simulink model "CF009A_GmOvrlStMgr"  (R2013b)
settings: Solver=FixedStepDiscrete  SolverMode=SingleTasking  StartTime=0.0  StopTime=1  FixedStep=0.002  RelTol=1e-3
values from neighbouring files (symbols this model uses):
  APASTACTV_CNT_U08 = DataDict.Constant    [CF009A_GmOvrlStMgr_DataDict.m]
  APASTCTRLAVL_CNT_U08 = DataDict.Constant    [CF009A_GmOvrlStMgr_DataDict.m]
  ARCHGLBPRM_2MILLISEC_SEC_F32 = DataDict.Constant    [CF009A_GmOvrlStMgr_DataDict.m]
  GmOvrlStMgrApaHwTqThd = DataDict.Calibration    [CF009A_GmOvrlStMgr_DataDict.m]
  GmOvrlStMgrApaHwTqTiThd = DataDict.Calibration    [CF009A_GmOvrlStMgr_DataDict.m]
  GmOvrlStMgrApaMfgEna = DataDict.Calibration    [CF009A_GmOvrlStMgr_DataDict.m]
  GmOvrlStMgrEscMfgEna = DataDict.Calibration    [CF009A_GmOvrlStMgr_DataDict.m]
  GmOvrlStMgrHaptcAmp = DataDict.Calibration    [CF009A_GmOvrlStMgr_DataDict.m]
  GmOvrlStMgrHaptcDurn = DataDict.Calibration    [CF009A_GmOvrlStMgr_DataDict.m]
  GmOvrlStMgrHaptcFrq = DataDict.Calibration    [CF009A_GmOvrlStMgr_DataDict.m]
  GmOvrlStMgrHaptcReactnTi = DataDict.Calibration    [CF009A_GmOvrlStMgr_DataDict.m]
  GmOvrlStMgrHaptcReqTiThd = DataDict.Calibration    [CF009A_GmOvrlStMgr_DataDict.m]
  GmOvrlStMgrHwAgTarLimr = DataDict.Calibration    [CF009A_GmOvrlStMgr_DataDict.m]
  GmOvrlStMgrLkaHwTqThd1 = DataDict.Calibration    [CF009A_GmOvrlStMgr_DataDict.m]
  GmOvrlStMgrLkaHwTqThd2 = DataDict.Calibration    [CF009A_GmOvrlStMgr_DataDict.m]
  GmOvrlStMgrLkaHwTqTiThd1 = DataDict.Calibration    [CF009A_GmOvrlStMgr_DataDict.m]
  GmOvrlStMgrLkaHwTqTiThd2 = DataDict.Calibration    [CF009A_GmOvrlStMgr_DataDict.m]
  GmOvrlStMgrLkaMfgEna = DataDict.Calibration    [CF009A_GmOvrlStMgr_DataDict.m]
  GmOvrlStMgrLoaMtgtnHaptcFbOffTi = DataDict.Calibration    [CF009A_GmOvrlStMgr_DataDict.m]
  GmOvrlStMgrLoaMtgtnHaptcFbOnTi = DataDict.Calibration    [CF009A_GmOvrlStMgr_DataDict.m]
  GmOvrlStMgrLoaMtgtnHaptcFbStrtOnTi = DataDict.Calibration    [CF009A_GmOvrlStMgr_DataDict.m]
  GmOvrlStMgrLoaMtgtnHaptcFbTqMax = DataDict.Calibration    [CF009A_GmOvrlStMgr_DataDict.m]
  GmOvrlStMgrLoaMtgtnHaptcFbTqMin = DataDict.Calibration    [CF009A_GmOvrlStMgr_DataDict.m]
  GmOvrlStMgrLoaMtgtnHaptcFbVehSpdMax = DataDict.Calibration    [CF009A_GmOvrlStMgr_DataDict.m]
  GmOvrlStMgrLoaMtgtnHaptcFbVehSpdMin = DataDict.Calibration    [CF009A_GmOvrlStMgr_DataDict.m]
  GmOvrlStMgrLoaMtgtnHaptcFrq = DataDict.Calibration    [CF009A_GmOvrlStMgr_DataDict.m]
  GmOvrlStMgrLoaMtgtnStrtHaptcAmp = DataDict.Calibration    [CF009A_GmOvrlStMgr_DataDict.m]
  GmOvrlStMgrLoaStIgnCntrThd = DataDict.Calibration    [CF009A_GmOvrlStMgr_DataDict.m]
  GmOvrlStMgrShiftLvrTiThd = DataDict.Calibration    [CF009A_GmOvrlStMgr_DataDict.m]
  GmOvrlStMgrStandStillThd = DataDict.Calibration    [CF009A_GmOvrlStMgr_DataDict.m]
  GmOvrlStMgrStandStillTiThd = DataDict.Calibration    [CF009A_GmOvrlStMgr_DataDict.m]
  HAPTCSTACTV_CNT_U08 = DataDict.Constant    [CF009A_GmOvrlStMgr_DataDict.m]
  HAPTCSTWAIT_CNT_U08 = DataDict.Constant    [CF009A_GmOvrlStMgr_DataDict.m]
  HWOSCNFRQMIN_HZ_F32 = DataDict.Constant    [CF009A_GmOvrlStMgr_DataDict.m]
  LKAFLTCNTRTHD_CNT_U08 = DataDict.Constant    [CF009A_GmOvrlStMgr_DataDict.m]
  LKAFLTTMRTHD_MILLISEC_U32 = DataDict.Constant    [CF009A_GmOvrlStMgr_DataDict.m]
  LKASTPRMNTFAILD_CNT_U08 = DataDict.Constant    [CF009A_GmOvrlStMgr_DataDict.m]
  LoaMtgtnThdExcdd = DataDict.NTC    [CF009A_GmOvrlStMgr_DataDict.m]
  MILLISECTO100MICROSECCNVN_CNT_U32 = DataDict.Constant    [CF009A_GmOvrlStMgr_DataDict.m]
  NODEBSTEP_CNT_U16 = DataDict.Constant    [CF009A_GmOvrlStMgr_DataDict.m]
undefined symbols (not defined in the file or in its folder): LoaSt1, NtcSts1, NVM_RequestResultType, SysSt1
libraries: simulink x13, Fil x6, NxtrNvM x4, NxtrLim x4, NxtrAbslt x3, NxtrSign x2, FixdToFloat x1, FloatToFixd x1, LnrIntrpn x1
(part 3 of 8)

== system CF009A_GmOvrlStMgr/GmOvrlStMgr/GmOvrlStMgrPer1/HwTqFildIntlChk ==
  In1 : Inport
  Abslt_f32_f32 : NxtrAbslt/Abslt_f32_f32  SFunctionSpec=single y1 = Abslt_f32_f32(single u1)
      settings: AttributesFormatString=%<Name>
  CopyRight2 : Subsystem  Description=|  mask(Copyright Information){none=on}
      | Copyright info block.                                               
      |                                                                     
      | Place copyright information at the top of every subsystem in design.
      mask prompts: none "No parameters"
      mask help: Place copyright information at the top of every subsystem in design.
      mask Display:
      | NxtrConf = 'Nexteer Confidential';
      | 
      | sys = bdroot; %handle for the current model ("system")
      | first = get_param(sys,'Created');
      | first = first(end-3:end);  %year is last four digits
      | 
      | last = get_param(sys,'LastModifiedDate');
      | if isempty(last)
      |     last = datestr(now,'yyyy');
      | else
      |     last = last(end-3:end);
      | end
      | 
      | if strcmp(first,last)
      |     fprintf('%s -- Copyright %s Nexteer',NxtrConf,first)
      | else
      |     fprintf('%s -- %s%s- %s Nexteer',NxtrConf,char(169),first,last)
      | end
  FilLpUpdOutp : Fil/FilLpUpdOutp  StVar=HwTqOscnLpFil
      settings: AttributesFormatString=StVar: %<StVar>
  Interval Test4 : simulink/Logic and Bit Operations/Interval Test  IntervalClosedRight=on  uplimit=GmOvrlStMgrLoaMtgtnHaptcFbTqMax  IntervalClosedLeft=on  lowlimit=GmOvrlStMgrLoaMtgtnHaptcFbTqMin  OutDataTypeStr=boolean
  Out1 : Outport
  wires:
  Interval Test4/1 -> Out1/1
  Abslt_f32_f32/1 -> Interval Test4/1
  FilLpUpdOutp/1 -> Abslt_f32_f32/1
  In1/1 -> FilLpUpdOutp/1

== system CF009A_GmOvrlStMgr/GmOvrlStMgr/GmOvrlStMgrPer1/Inct_IgnCntr_Once ==
  IgnCntrLcl : Inport  RequirementInfo={} %GIDa_31be0032_d248_4158_b577_634f04f9b9d9
  Action Port : ActionPort  ActionType=then
  CopyRight2 : Subsystem  Description=|  mask(Copyright Information){none=on}
      | Copyright info block.                                               
      |                                                                     
      | Place copyright information at the top of every subsystem in design.
      mask prompts: none "No parameters"
      mask help: Place copyright information at the top of every subsystem in design.
      mask Display:
      | NxtrConf = 'Nexteer Confidential';
      | 
      | sys = bdroot; %handle for the current model ("system")
      | first = get_param(sys,'Created');
      | if(isempty(first))
      |     first = datestr(now,'yyyy');
      | else
      |     first = first(end-3:end);  %year is last four digits
      | end
      | 
      | last = get_param(sys,'LastModifiedDate');
      | if isempty(last)
      |     last = datestr(now,'yyyy');
      | else
      |     last = last(end-3:end);
      | end
      | 
      | if strcmp(first,last)
      |     fprintf('%s -- Copyright %s Nexteer',NxtrConf,first)
      | else
      |     fprintf('%s -- %s%s- %s Nexteer',NxtrConf,char(169),first,last)
      | end
  Data Store Read1 : DataStoreRead  DataStoreName=IgnCntrUpd
  If20 : If  IfExpression=~u1  ShowElse=off
  IgnCntr : Subsystem  TreatAsAtomicUnit=on
  wires:
  If20/1 -> IgnCntr/Action
  Data Store Read1/1 -> If20/1
  IgnCntrLcl/1 -> IgnCntr/1(IgnCntrLcl)

== system CF009A_GmOvrlStMgr/GmOvrlStMgr/GmOvrlStMgrPer1/LKAIntv ==
  note: To Determine if the driver is opposing the LKA command
  HwTq : Inport
  LkaTqCmdCdnd : Inport  Port=2
  Abslt_f32_f32 : NxtrAbslt/Abslt_f32_f32  SFunctionSpec=single y1 = Abslt_f32_f32(single u1)
      settings: AttributesFormatString=%<Name>
  CopyRight2 : Subsystem  Description=|  mask(Copyright Information){none=on}
      | Copyright info block.                                               
      |                                                                     
      | Place copyright information at the top of every subsystem in design.
      mask prompts: none "No parameters"
      mask help: Place copyright information at the top of every subsystem in design.
      mask Display:
      | NxtrConf = 'Nexteer Confidential';
      | 
      | sys = bdroot; %handle for the current model ("system")
      | first = get_param(sys,'Created');
      | first = first(end-3:end);  %year is last four digits
      | 
      | last = get_param(sys,'LastModifiedDate');
      | if isempty(last)
      |     last = datestr(now,'yyyy');
      | else
      |     last = last(end-3:end);
      | end
      | 
      | if strcmp(first,last)
      |     fprintf('%s -- Copyright %s Nexteer',NxtrConf,first)
      | else
      |     fprintf('%s -- %s%s- %s Nexteer',NxtrConf,char(169),first,last)
      | end
  Data Store Write1 : DataStoreWrite  DataStoreName=LkaIntvPrev
  FilLpUpdOutp : Fil/FilLpUpdOutp  StVar=HwTqLkaLpFil
      settings: AttributesFormatString=StVar: %<StVar>
  HwTqLkaTqSignEqu : Subsystem  TreatAsAtomicUnit=on
  HwTqLkaTqSignNotEqu : Subsystem  TreatAsAtomicUnit=on
  If2 : If  IfExpression=u1
  Merge3 : Merge
  Relational Operator : RelationalOperator  Operator===  OutDataTypeStr=boolean
  Sign_s08_f1 : NxtrSign/Sign_s08_f32  SFunctionSpec=int8 y1 = Sign_s08_f32(single u1)
  Sign_s08_f32 : NxtrSign/Sign_s08_f32  SFunctionSpec=int8 y1 = Sign_s08_f32(single u1)
  LKAIntv : Outport
  wires:
  [HwTq] -> Sign_s08_f1/1
  FilLpUpdOutp/1 -> Abslt_f32_f32/1
  LkaTqCmdCdnd/1 -> Sign_s08_f32/1
  Sign_s08_f32/1 -> Relational Operator/2
  Sign_s08_f1/1 -> Relational Operator/1
  Relational Operator/1 -> If2/1
  If2/1 -> HwTqLkaTqSignEqu/Action
  If2/2 -> HwTqLkaTqSignNotEqu/Action
  Abslt_f32_f32/1 -> [AbsHwTqFild]
  HwTq/1 -> [HwTq], FilLpUpdOutp/1
  [AbsHwTqFild] -> HwTqLkaTqSignNotEqu/1(AbsHwTqFild)
  HwTqLkaTqSignEqu/1(LKAIntv) -> Merge3/1
  HwTqLkaTqSignNotEqu/1(LKAIntv) -> Merge3/2
  Merge3/1 -> Data Store Write1/1, LKAIntv/1

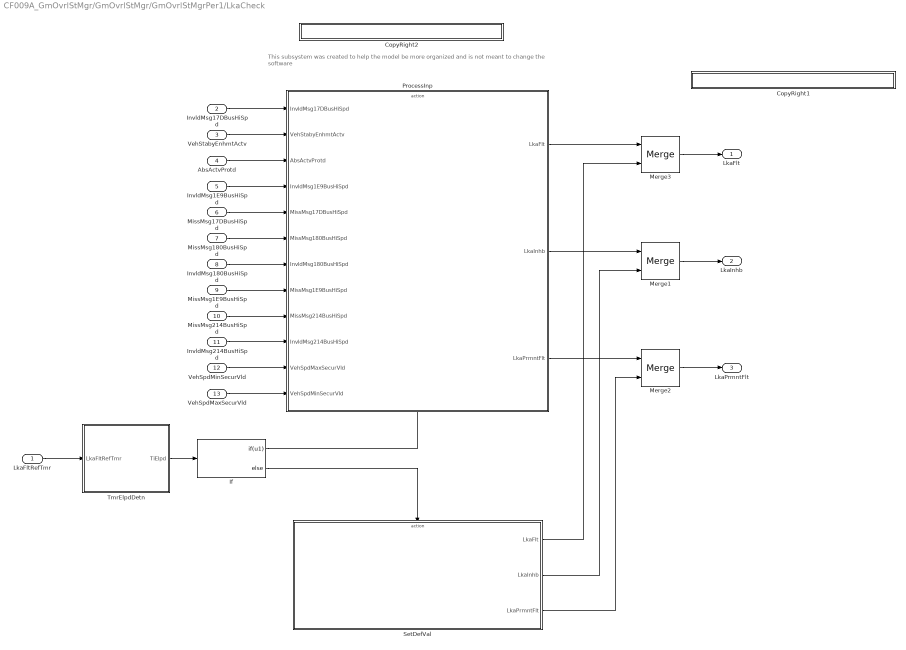
== system CF009A_GmOvrlStMgr/GmOvrlStMgr/GmOvrlStMgrPer1/LkaCheck ==
  note: This subsystem was created to help the model be more organized and is not meant to change the software
  LkaFltRefTmr : Inport
  InvldMsg17DBusHiSpd : Inport  RequirementInfo={} %GIDa_2e808d10_eb15_4dce_ab7e_f3136c3c94f9  Port=2
  VehStabyEnhmtActv : Inport  RequirementInfo={} %GIDa_3591af50_b788_48cc_aa03_0dae07c6844d  Port=3
  AbsActvProtd : Inport  RequirementInfo={} %GIDa_a71630fb_1116_4598_9016_42ba8f18e277  Port=4
  InvldMsg1E9BusHiSpd : Inport  RequirementInfo={} %GIDa_44549ea5_d3bf_44aa_ad01_370864df879b  Port=5
  MissMsg17DBusHiSpd : Inport  RequirementInfo={} %GIDa_3510a1c9_681a_4837_901b_d1fdb7257903  Port=6
  MissMsg180BusHiSpd : Inport  RequirementInfo={} %GIDa_29db47c2_2496_45a5_a94f_ca81858af381  Port=7
  InvldMsg180BusHiSpd : Inport  RequirementInfo={} %GIDa_c95a73a8_1984_48d0_982e_2a99b56d2733  Port=8
  MissMsg1E9BusHiSpd : Inport  RequirementInfo={} %GIDa_8896b252_879d_4242_80a0_160e6dd0973f  Port=9
  MissMsg214BusHiSpd : Inport  RequirementInfo={} %GIDa_e93b804e_26b6_4a26_9fbc_29131c435554  Port=10
  InvldMsg214BusHiSpd : Inport  RequirementInfo={} %GIDa_23b949d5_a203_4809_9d67_db82e22a32ce  Port=11
  VehSpdMinSecurVld : Inport  Port=12
  VehSpdMaxSecurVld : Inport  Port=13
  CopyRight1 : Subsystem  Description=|  mask(Copyright Information){none=on}
      | Copyright info block.                                               
      |                                                                     
      | Place copyright information at the top of every subsystem in design.
      mask prompts: none "No parameters"
      mask help: Place copyright information at the top of every subsystem in design.
      mask Display:
      | NxtrConf = 'Nexteer Confidential';
      | 
      | sys = bdroot; %handle for the current model ("system")
      | first = get_param(sys,'Created');
      | if(isempty(first))
      |     first = datestr(now,'yyyy');
      | else
      |     first = first(end-3:end);  %year is last four digits
      | end
      | 
      | last = get_param(sys,'LastModifiedDate');
      | if isempty(last)
      |     last = datestr(now,'yyyy');
      | else
      |     last = last(end-3:end);
      | end
      | 
      | if strcmp(first,last)
      |     fprintf('%s -- Copyright %s Nexteer',NxtrConf,first)
      | else
      |     fprintf('%s -- %s%s- %s Nexteer',NxtrConf,char(169),first,last)
      | end
  CopyRight2 : Subsystem  Description=|  mask(Copyright Information){none=on}
      | Copyright info block.                                               
      |                                                                     
      | Place copyright information at the top of every subsystem in design.
      mask prompts: none "No parameters"
      mask help: Place copyright information at the top of every subsystem in design.
      mask Display:
      | NxtrConf = 'Nexteer Confidential';
      | 
      | sys = bdroot; %handle for the current model ("system")
      | first = get_param(sys,'Created');
      | first = first(end-3:end);  %year is last four digits
      | 
      | last = get_param(sys,'LastModifiedDate');
      | if isempty(last)
      |     last = datestr(now,'yyyy');
      | else
      |     last = last(end-3:end);
      | end
      | 
      | if strcmp(first,last)
      |     fprintf('%s -- Copyright %s Nexteer',NxtrConf,first)
      | else
      |     fprintf('%s -- %s%s- %s Nexteer',NxtrConf,char(169),first,last)
      | end
  If : If  RequirementInfo={} %GIDa_1f091b25_2844_4bea_86d8_428600b90772  Priority=0  IfExpression=u1
  Merge1 : Merge  RequirementInfo={} %GIDa_91ec1541_edd6_4e63_a334_a58d5e1b75c9
  Merge2 : Merge  RequirementInfo={} %GIDa_1f0d8a4f_5d48_411b_8451_0a42805f8c5f
  Merge3 : Merge  RequirementInfo={} %GIDa_d55ab1e5_a42e_4154_95a8_1fe89e6aae2d
  ProcessInp : Subsystem  TreatAsAtomicUnit=on
  SetDefVal : Subsystem  TreatAsAtomicUnit=on
  TmrElpdDetn : Subsystem  RequirementInfo={} %GIDa_14aacf7e_b947_4f82_958b_883fcdf93c59  TreatAsAtomicUnit=on
  LkaFlt : Outport
  LkaInhb : Outport  Port=2
  LkaPrmntFlt : Outport  Port=3
  wires:
  LkaFltRefTmr/1 -> TmrElpdDetn/1(LkaFltRefTmr)
  TmrElpdDetn/1(TiElpd) -> If/1
  If/2 -> SetDefVal/Action
  If/1 -> ProcessInp/Action
  MissMsg17DBusHiSpd/1 -> ProcessInp/5(MissMsg17DBusHiSpd)
  MissMsg180BusHiSpd/1 -> ProcessInp/6(MissMsg180BusHiSpd)
  InvldMsg180BusHiSpd/1 -> ProcessInp/7(InvldMsg180BusHiSpd)
  MissMsg1E9BusHiSpd/1 -> ProcessInp/8(MissMsg1E9BusHiSpd)
  MissMsg214BusHiSpd/1 -> ProcessInp/9(MissMsg214BusHiSpd)
  InvldMsg214BusHiSpd/1 -> ProcessInp/10(InvldMsg214BusHiSpd)
  VehSpdMinSecurVld/1 -> ProcessInp/11(VehSpdMaxSecurVld)
  VehSpdMaxSecurVld/1 -> ProcessInp/12(VehSpdMinSecurVld)
  InvldMsg17DBusHiSpd/1 -> ProcessInp/1(InvldMsg17DBusHiSpd)
  VehStabyEnhmtActv/1 -> ProcessInp/2(VehStabyEnhmtActv)
  AbsActvProtd/1 -> ProcessInp/3(AbsActvProtd)
  InvldMsg1E9BusHiSpd/1 -> ProcessInp/4(InvldMsg1E9BusHiSpd)
  ProcessInp/1(LkaFlt) -> Merge3/1
  Merge3/1 -> LkaFlt/1
  Merge1/1 -> LkaInhb/1
  Merge2/1 -> LkaPrmntFlt/1
  SetDefVal/1(LkaFlt) -> Merge3/2
  ProcessInp/2(LkaInhb) -> Merge1/1
  SetDefVal/2(LkaInhb) -> Merge1/2
  ProcessInp/3(LkaPrmntFlt) -> Merge2/1
  SetDefVal/3(LkaPrmntFlt) -> Merge2/2

== system CF009A_GmOvrlStMgr/GmOvrlStMgr/GmOvrlStMgrPer1/LoaStLimdOrSwBasdMtgtn ==
  LoaSt : Inport
  CopyRight2 : Subsystem  Description=|  mask(Copyright Information){none=on}
      | Copyright info block.                                               
      |                                                                     
      | Place copyright information at the top of every subsystem in design.
      mask prompts: none "No parameters"
      mask help: Place copyright information at the top of every subsystem in design.
      mask Display:
      | NxtrConf = 'Nexteer Confidential';
      | 
      | sys = bdroot; %handle for the current model ("system")
      | first = get_param(sys,'Created');
      | if(isempty(first))
      |     first = datestr(now,'yyyy');
      | else
      |     first = first(end-3:end);  %year is last four digits
      | end
      | 
      | last = get_param(sys,'LastModifiedDate');
      | if isempty(last)
      |     last = datestr(now,'yyyy');
      | else
      |     last = last(end-3:end);
      | end
      | 
      | if strcmp(first,last)
      |     fprintf('%s -- Copyright %s Nexteer',NxtrConf,first)
      | else
      |     fprintf('%s -- %s%s- %s Nexteer',NxtrConf,char(169),first,last)
      | end
  Enumerated Constant : simulink/Sources/Enumerated Constant  OutDataTypeStr=Enum: LoaSt1  Value=LoaSt1.LOAST_LIMD  SampleTime=inf
  Enumerated Constant1 : simulink/Sources/Enumerated Constant  OutDataTypeStr=Enum: LoaSt1  Value=LoaSt1.LOAST_SWBASDMTGTN  SampleTime=inf
  If2 : If  IfExpression=u1
  Logical Operator5 : Logic  Operator=OR  AllPortsSameDT=off  OutDataTypeStr=boolean
  Merge : Merge
  Relational Operator2 : RelationalOperator  Operator===  OutDataTypeStr=boolean
  Relational Operator4 : RelationalOperator  Operator===  OutDataTypeStr=boolean
  Set_false_LoaStLimdOrSwBasdMtgtn : Subsystem
  Set_true_LoaStLimdOrSwBasdMtgtn : Subsystem
  LoaStLimdOrSwBasdMtgtn : Outport
  wires:
  Set_true_LoaStLimdOrSwBasdMtgtn/1(LoaStLimdOrSwBasdMtgtn) -> Merge/1
  If2/1 -> Set_true_LoaStLimdOrSwBasdMtgtn/Action
  Relational Operator4/1 -> Logical Operator5/2
  Enumerated Constant/1 -> Relational Operator2/1
  If2/2 -> Set_false_LoaStLimdOrSwBasdMtgtn/Action
  Enumerated Constant1/1 -> Relational Operator4/2
  LoaSt/1 -> Relational Operator4/1, Relational Operator2/2
  Logical Operator5/1 -> If2/1
  Relational Operator2/1 -> Logical Operator5/1
  Set_false_LoaStLimdOrSwBasdMtgtn/1(LoaStLimdOrSwBasdMtgtn) -> Merge/2
  Merge/1 -> LoaStLimdOrSwBasdMtgtn/1

== system CF009A_GmOvrlStMgr/GmOvrlStMgr/GmOvrlStMgrPer1/SysStNotOperate_TqOscnDi_AmpZero_FrqMin ==
  Action Port : ActionPort  ActionType=else
  Constant : Constant  Value=0  OutDataTypeStr=single
  Constant1 : Constant  Value=HWOSCNFRQMIN_HZ_F32  OutDataTypeStr=single
  Constant9 : Constant  Value=false  OutDataTypeStr=boolean
      settings: AttributesFormatString=%<OutDataTypeStr>
  CopyRight2 : Subsystem  Description=|  mask(Copyright Information){none=on}
      | Copyright info block.                                               
      |                                                                     
      | Place copyright information at the top of every subsystem in design.
      mask prompts: none "No parameters"
      mask help: Place copyright information at the top of every subsystem in design.
      mask Display:
      | NxtrConf = 'Nexteer Confidential';
      | 
      | sys = bdroot; %handle for the current model ("system")
      | first = get_param(sys,'Created');
      | if(isempty(first))
      |     first = datestr(now,'yyyy');
      | else
      |     first = first(end-3:end);  %year is last four digits
      | end
      | 
      | last = get_param(sys,'LastModifiedDate');
      | if isempty(last)
      |     last = datestr(now,'yyyy');
      | else
      |     last = last(end-3:end);
      | end
      | 
      | if strcmp(first,last)
      |     fprintf('%s -- Copyright %s Nexteer',NxtrConf,first)
      | else
      |     fprintf('%s -- %s%s- %s Nexteer',NxtrConf,char(169),first,last)
      | end
  HwOscnEna : Outport  RequirementInfo={} %GIDa_8ea3e658_ac34_4ba8_8bc0_f59fa217fe1b
  HwOscnMotAmp : Outport  RequirementInfo={} %GIDa_cab656c5_ad5b_40cd_9e56_00ba20adb2b9  Port=2
  HwOscnFrq : Outport  RequirementInfo={} %GIDa_8a1cbf52_fe7e_4d9e_a07e_11d275854390  Port=3
  wires:
  Constant9/1 -> HwOscnEna/1
  Constant/1 -> HwOscnMotAmp/1
  Constant1/1 -> HwOscnFrq/1

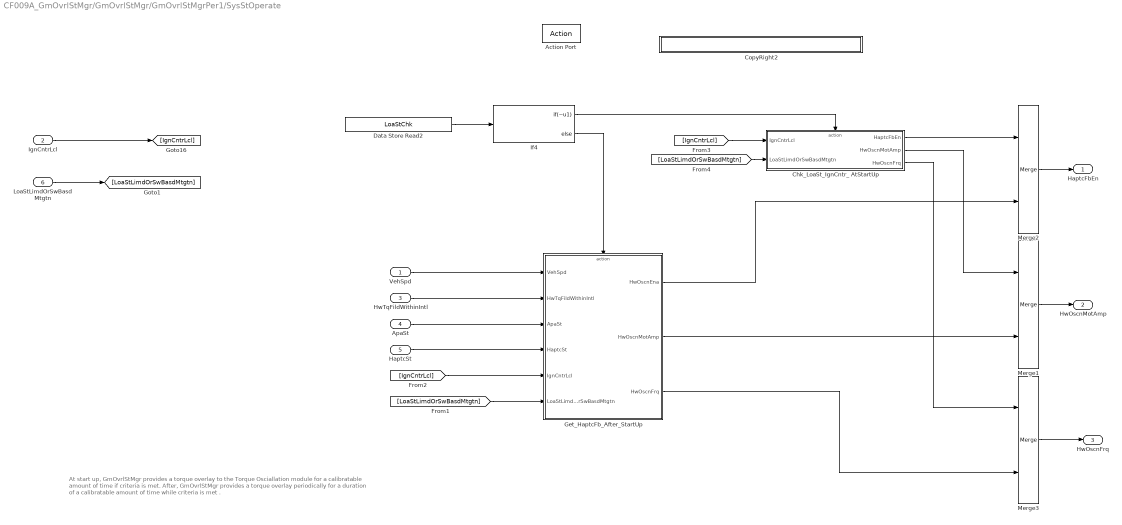
== system CF009A_GmOvrlStMgr/GmOvrlStMgr/GmOvrlStMgrPer1/SysStOperate ==
  note: At start up, GmOvrlStMgr provides a torque overlay to the Torque Osciallation module for a calibratable amount of time if criteria is met.
      | After, GmOvrlStMgr provides a torque overlay periodically for a duration of a calibratable amount of time while criteria is met .
  VehSpd : Inport  RequirementInfo={} %GIDa_2652915f_2b3a_4256_8b6a_592e4995acc0
  IgnCntrLcl : Inport  RequirementInfo={} %GIDa_e888d205_558d_4af3_99a0_723aa084dc2d  Port=2
  HwTqFildWithinIntl : Inport  RequirementInfo={} %GIDa_45987a6d_ef79_4fe8_8691_cf583e52523b  Port=3
  ApaSt : Inport  RequirementInfo={} %GIDa_af2c68b1_95b1_4974_8eec_dffb9414db10  Port=4
  HaptcSt : Inport  RequirementInfo={} %GIDa_9d2ea291_f891_4713_85e4_8f6b9ae44dd1  Port=5
  LoaStLimdOrSwBasdMtgtn : Inport  RequirementInfo={} %GIDa_9e2f6aad_f776_44c0_8c0b_e29e77d1c4aa  Port=6
  Action Port : ActionPort  ActionType=then
  Chk_LoaSt_IgnCntr_ AtStartUp : Subsystem  TreatAsAtomicUnit=on
  CopyRight2 : Subsystem  Description=|  mask(Copyright Information){none=on}
      | Copyright info block.                                               
      |                                                                     
      | Place copyright information at the top of every subsystem in design.
      mask prompts: none "No parameters"
      mask help: Place copyright information at the top of every subsystem in design.
      mask Display:
      | NxtrConf = 'Nexteer Confidential';
      | 
      | sys = bdroot; %handle for the current model ("system")
      | first = get_param(sys,'Created');
      | if(isempty(first))
      |     first = datestr(now,'yyyy');
      | else
      |     first = first(end-3:end);  %year is last four digits
      | end
      | 
      | last = get_param(sys,'LastModifiedDate');
      | if isempty(last)
      |     last = datestr(now,'yyyy');
      | else
      |     last = last(end-3:end);
      | end
      | 
      | if strcmp(first,last)
      |     fprintf('%s -- Copyright %s Nexteer',NxtrConf,first)
      | else
      |     fprintf('%s -- %s%s- %s Nexteer',NxtrConf,char(169),first,last)
      | end
  Data Store Read2 : DataStoreRead  DataStoreName=LoaStChk
  Get_HaptcFb_After_StartUp : Subsystem  TreatAsAtomicUnit=on
  If4 : If  IfExpression=~u1
  Merge1 : Merge
  Merge2 : Merge
  Merge3 : Merge
  HaptcFbEn : Outport
  HwOscnMotAmp : Outport  RequirementInfo={} %GIDa_30e263ba_ec21_46fb_a2a6_c50359a0704f  Port=2
  HwOscnFrq : Outport  RequirementInfo={} %GIDa_0a2b2e9b_0783_462d_9074_6b0e98e66f91  Port=3
  wires:
  Data Store Read2/1 -> If4/1
  If4/1 -> Chk_LoaSt_IgnCntr_ AtStartUp/Action
  If4/2 -> Get_HaptcFb_After_StartUp/Action
  Chk_LoaSt_IgnCntr_ AtStartUp/2(HwOscnMotAmp) -> Merge1/1
  Chk_LoaSt_IgnCntr_ AtStartUp/1(HaptcFbEn) -> Merge2/1
  Chk_LoaSt_IgnCntr_ AtStartUp/3(HwOscnFrq) -> Merge3/1
  Get_HaptcFb_After_StartUp/1(HwOscnEna) -> Merge2/2
  Get_HaptcFb_After_StartUp/3(HwOscnFrq) -> Merge3/2
  Get_HaptcFb_After_StartUp/2(HwOscnMotAmp) -> Merge1/2
  Merge2/1 -> HaptcFbEn/1
  Merge3/1 -> HwOscnFrq/1
  Merge1/1 -> HwOscnMotAmp/1
  VehSpd/1 -> Get_HaptcFb_After_StartUp/1(VehSpd)
  HwTqFildWithinIntl/1 -> Get_HaptcFb_After_StartUp/2(HwTqFildWithinIntl)
  ApaSt/1 -> Get_HaptcFb_After_StartUp/3(ApaSt)
  HaptcSt/1 -> Get_HaptcFb_After_StartUp/4(HaptcSt)
  IgnCntrLcl/1 -> [IgnCntrLcl]
  [IgnCntrLcl] -> Chk_LoaSt_IgnCntr_ AtStartUp/1(IgnCntrLcl)
  [IgnCntrLcl] -> Get_HaptcFb_After_StartUp/5(IgnCntrLcl)
  [LoaStLimdOrSwBasdMtgtn] -> Get_HaptcFb_After_StartUp/6(LoaStLimdOrSwBasdMtgtn)
  LoaStLimdOrSwBasdMtgtn/1 -> [LoaStLimdOrSwBasdMtgtn]
  [LoaStLimdOrSwBasdMtgtn] -> Chk_LoaSt_IgnCntr_ AtStartUp/2(LoaStLimdOrSwBasdMtgtn)

== system CF009A_GmOvrlStMgr/GmOvrlStMgr/GmOvrlStMgrPer1/Timer for HwHaptcEna ==
  Ena : Inport
  TiThd : Inport  Port=2
  Constant : Constant  Value=0  OutDataTypeStr=uint32
  Constant2 : Constant  Value=MILLISECTO100MICROSECCNVN_CNT_U32
  CopyRight2 : Subsystem  Description=|  mask(Copyright Information){none=on}
      | Copyright info block.                                               
      |                                                                     
      | Place copyright information at the top of every subsystem in design.
      mask prompts: none "No parameters"
      mask help: Place copyright information at the top of every subsystem in design.
      mask Display:
      | NxtrConf = 'Nexteer Confidential';
      | 
      | sys = bdroot; %handle for the current model ("system")
      | first = get_param(sys,'Created');
      | if(isempty(first))
      |     first = datestr(now,'yyyy');
      | else
      |     first = first(end-3:end);  %year is last four digits
      | end
      | 
      | last = get_param(sys,'LastModifiedDate');
      | if isempty(last)
      |     last = datestr(now,'yyyy');
      | else
      |     last = last(end-3:end);
      | end
      | 
      | if strcmp(first,last)
      |     fprintf('%s -- Copyright %s Nexteer',NxtrConf,first)
      | else
      |     fprintf('%s -- %s%s- %s Nexteer',NxtrConf,char(169),first,last)
      | end
  Data Store Read : DataStoreRead  Priority=1  DataStoreName=PrevHaptcReqEna
      settings: AttributesFormatString="Priority:  %<Priority>"
  Data Store Write1 : DataStoreWrite  Priority=2  DataStoreName=PrevHaptcReqEna
      settings: AttributesFormatString="Priority:  %<Priority>"
  If : If  NumInputs=2  IfExpression=u1&(~u2)  ElseIfExpressions=u1&u2
  If Action Subsystem : Subsystem  TreatAsAtomicUnit=on
  If Action Subsystem1 : Subsystem  TreatAsAtomicUnit=on
  If Action Subsystem2 : Subsystem  TreatAsAtomicUnit=on
  Merge : Merge  Inputs=3
  Product : Product
  Relational Operator3 : RelationalOperator  OutDataTypeStr=boolean
  Out1 : Outport
  wires:
  If Action Subsystem2/1(Out1) -> Merge/2
  If/2 -> If Action Subsystem2/Action
  Data Store Read/1 -> If/2
  Ena/1 -> If/1, Data Store Write1/1
  Relational Operator3/1 -> Out1/1
  Merge/1 -> Relational Operator3/1
  Product/1 -> Relational Operator3/2
  Constant2/1 -> Product/2
  TiThd/1 -> Product/1
  Constant/1 -> If Action Subsystem1/1(In1)
  If Action Subsystem1/1(Out1) -> Merge/3
  If Action Subsystem/1(Out) -> Merge/1
  If/3 -> If Action Subsystem1/Action
  If/1 -> If Action Subsystem/Action

== system CF009A_GmOvrlStMgr/GmOvrlStMgr/GmOvrlStMgrPer1/Timer for ShiftLvrRvs ==
  Ena : Inport
  TiThd : Inport  Port=2
  Constant : Constant  Value=0  OutDataTypeStr=uint32
  Constant2 : Constant  Value=MILLISECTO100MICROSECCNVN_CNT_U32
  CopyRight2 : Subsystem  Description=|  mask(Copyright Information){none=on}
      | Copyright info block.                                               
      |                                                                     
      | Place copyright information at the top of every subsystem in design.
      mask prompts: none "No parameters"
      mask help: Place copyright information at the top of every subsystem in design.
      mask Display:
      | NxtrConf = 'Nexteer Confidential';
      | 
      | sys = bdroot; %handle for the current model ("system")
      | first = get_param(sys,'Created');
      | first = first(end-3:end);  %year is last four digits
      | 
      | last = get_param(sys,'LastModifiedDate');
      | if isempty(last)
      |     last = datestr(now,'yyyy');
      | else
      |     last = last(end-3:end);
      | end
      | 
      | if strcmp(first,last)
      |     fprintf('%s -- Copyright %s Nexteer',NxtrConf,first)
      | else
      |     fprintf('%s -- %s%s- %s Nexteer',NxtrConf,char(169),first,last)
      | end
  Data Store Read : DataStoreRead  Priority=1  DataStoreName=PrevShiftLvrRvsEna
      settings: AttributesFormatString="priority:  %<Priority>"
  Data Store Write1 : DataStoreWrite  Priority=2  DataStoreName=PrevShiftLvrRvsEna
      settings: AttributesFormatString="priority:  %<Priority>"
  If : If  NumInputs=2  IfExpression=u1&(~u2)  ElseIfExpressions=u1&u2
  If Action Subsystem : Subsystem  TreatAsAtomicUnit=on
  If Action Subsystem1 : Subsystem  TreatAsAtomicUnit=on
  If Action Subsystem2 : Subsystem  TreatAsAtomicUnit=on
  Merge : Merge  Inputs=3
  Product : Product
  Relational Operator3 : RelationalOperator  OutDataTypeStr=boolean
  Out1 : Outport
  wires:
  If Action Subsystem2/1(Out) -> Merge/2
  If/2 -> If Action Subsystem2/Action
  Data Store Read/1 -> If/2
  Ena/1 -> If/1, Data Store Write1/1
  Relational Operator3/1 -> Out1/1
  Merge/1 -> Relational Operator3/1
  Product/1 -> Relational Operator3/2
  Constant2/1 -> Product/2
  TiThd/1 -> Product/1
  Constant/1 -> If Action Subsystem1/1(In1)
  If Action Subsystem1/1(Out1) -> Merge/3
  If Action Subsystem/1(Out) -> Merge/1
  If/3 -> If Action Subsystem1/Action
  If/1 -> If Action Subsystem/Action

== system CF009A_GmOvrlStMgr/GmOvrlStMgr/GmOvrlStMgrPer1/Timer for VehStandStill ==
  Ena : Inport
  TiThd : Inport  Port=2
  Constant : Constant  Value=0  OutDataTypeStr=uint32
  Constant2 : Constant  Value=MILLISECTO100MICROSECCNVN_CNT_U32
  CopyRight2 : Subsystem  Description=|  mask(Copyright Information){none=on}
      | Copyright info block.                                               
      |                                                                     
      | Place copyright information at the top of every subsystem in design.
      mask prompts: none "No parameters"
      mask help: Place copyright information at the top of every subsystem in design.
      mask Display:
      | NxtrConf = 'Nexteer Confidential';
      | 
      | sys = bdroot; %handle for the current model ("system")
      | first = get_param(sys,'Created');
      | first = first(end-3:end);  %year is last four digits
      | 
      | last = get_param(sys,'LastModifiedDate');
      | if isempty(last)
      |     last = datestr(now,'yyyy');
      | else
      |     last = last(end-3:end);
      | end
      | 
      | if strcmp(first,last)
      |     fprintf('%s -- Copyright %s Nexteer',NxtrConf,first)
      | else
      |     fprintf('%s -- %s%s- %s Nexteer',NxtrConf,char(169),first,last)
      | end
  Data Store Read : DataStoreRead  Priority=1  DataStoreName=PrevVehStandStillEna
      settings: AttributesFormatString="Priority:  %<Priority>"
  Data Store Write1 : DataStoreWrite  Priority=2  DataStoreName=PrevVehStandStillEna
      settings: AttributesFormatString="Priority:  %<Priority>"
  If : If  NumInputs=2  IfExpression=u1&(~u2)  ElseIfExpressions=u1&u2
  If Action Subsystem : Subsystem  TreatAsAtomicUnit=on
  If Action Subsystem1 : Subsystem  TreatAsAtomicUnit=on
  If Action Subsystem2 : Subsystem  TreatAsAtomicUnit=on
  Merge : Merge  Inputs=3
  Product : Product
  Relational Operator3 : RelationalOperator  OutDataTypeStr=boolean
  Out1 : Outport
  wires:
  If Action Subsystem2/1(Out1) -> Merge/2
  If/2 -> If Action Subsystem2/Action
  Data Store Read/1 -> If/2
  Ena/1 -> If/1, Data Store Write1/1
  Relational Operator3/1 -> Out1/1
  Merge/1 -> Relational Operator3/1
  Product/1 -> Relational Operator3/2
  Constant2/1 -> Product/2
  TiThd/1 -> Product/1
  Constant/1 -> If Action Subsystem1/1(In1)
  If Action Subsystem1/1(Out1) -> Merge/3
  If Action Subsystem/1(Out) -> Merge/1
  If/3 -> If Action Subsystem1/Action
  If/1 -> If Action Subsystem/Action

== system CF009A_GmOvrlStMgr/GmOvrlStMgr/GmOvrlStMgrPer1/TransHaptcsWaitToAPAStActvFlg ==
  In1 : Inport
  In2 : Inport  Port=2
  CopyRight2 : Subsystem  Description=|  mask(Copyright Information){none=on}
      | Copyright info block.                                               
      |                                                                     
      | Place copyright information at the top of every subsystem in design.
      mask prompts: none "No parameters"
      mask help: Place copyright information at the top of every subsystem in design.
      mask Display:
      | NxtrConf = 'Nexteer Confidential';
      | 
      | sys = bdroot; %handle for the current model ("system")
      | first = get_param(sys,'Created');
      | first = first(end-3:end);  %year is last four digits
      | 
      | last = get_param(sys,'LastModifiedDate');
      | if isempty(last)
      |     last = datestr(now,'yyyy');
      | else
      |     last = last(end-3:end);
      | end
      | 
      | if strcmp(first,last)
      |     fprintf('%s -- Copyright %s Nexteer',NxtrConf,first)
      | else
      |     fprintf('%s -- %s%s- %s Nexteer',NxtrConf,char(169),first,last)
      | end
  ElpseTi : Subsystem
  If1 : If  NumInputs=2  IfExpression=u1&u2
  Merge3 : Merge
  RefTi : Subsystem
  Out1 : Outport
  wires:
  In1/1 -> If1/1
  If1/1 -> ElpseTi/Action
  If1/2 -> RefTi/Action
  ElpseTi/1(Out1) -> Merge3/1
  RefTi/1(Out1) -> Merge3/2
  Merge3/1 -> Out1/1
  In2/1 -> If1/2

== system CF009A_GmOvrlStMgr/GmOvrlStMgr/SetGmLoaIgnCntr/CopyRight2 ==

== system CF009A_GmOvrlStMgr/GmOvrlStMgr/GmOvrlStMgrInit1/GetRefTmr100MicroSec32bit/CopyRight2 ==

== system CF009A_GmOvrlStMgr/GmOvrlStMgr/GmOvrlStMgrInit1/NTC_Fault1_Set_Faild/SetNtcSts ==
  NtcNr : Inport
  NtcStInfo : Inport  Port=2
  NtcSts : Inport  Port=3
  DebStep : Inport  Port=4
  CopyRight2 : Subsystem  Description=|  mask(Copyright Information){none=on}
      | Copyright info block.                                               
      |                                                                     
      | Place copyright information at the top of every subsystem in design.
      mask prompts: none "No parameters"
      mask help: Place copyright information at the top of every subsystem in design.
      mask Display:
      | NxtrConf = 'Nexteer Confidential';
      | 
      | sys = bdroot; %handle for the current model ("system")
      | first = get_param(sys,'Created');
      | first = first(end-3:end);  %year is last four digits
      | 
      | last = get_param(sys,'LastModifiedDate');
      | if isempty(last)
      |     last = datestr(now,'yyyy');
      | else
      |     last = last(end-3:end);
      | end
      | 
      | if strcmp(first,last)
      |     fprintf('%s -- Copyright %s Nexteer',NxtrConf,first)
      | else
      |     fprintf('%s -- %s%s- %s Nexteer',NxtrConf,char(169),first,last)
      | end
  Data Store Write3 : DataStoreWrite  DataStoreName=Fault1_Status
  Terminator : Terminator
  Terminator1 : Terminator
  Terminator2 : Terminator
  wires:
  DebStep/1 -> Terminator2/1
  NtcSts/1 -> Data Store Write3/1
  NtcNr/1 -> Terminator/1
  NtcStInfo/1 -> Terminator1/1

== system CF009A_GmOvrlStMgr/GmOvrlStMgr/GmOvrlStMgrInit1/NTC_Fault1_Set_Passd/SetNtcSts ==
  NtcNr : Inport
  NtcStInfo : Inport  Port=2
  NtcSts : Inport  Port=3
  DebStep : Inport  Port=4
  CopyRight2 : Subsystem  Description=|  mask(Copyright Information){none=on}
      | Copyright info block.                                               
      |                                                                     
      | Place copyright information at the top of every subsystem in design.
      mask prompts: none "No parameters"
      mask help: Place copyright information at the top of every subsystem in design.
      mask Display:
      | NxtrConf = 'Nexteer Confidential';
      | 
      | sys = bdroot; %handle for the current model ("system")
      | first = get_param(sys,'Created');
      | first = first(end-3:end);  %year is last four digits
      | 
      | last = get_param(sys,'LastModifiedDate');
      | if isempty(last)
      |     last = datestr(now,'yyyy');
      | else
      |     last = last(end-3:end);
      | end
      | 
      | if strcmp(first,last)
      |     fprintf('%s -- Copyright %s Nexteer',NxtrConf,first)
      | else
      |     fprintf('%s -- %s%s- %s Nexteer',NxtrConf,char(169),first,last)
      | end
  Data Store Write3 : DataStoreWrite  DataStoreName=Fault1_Status
  Terminator : Terminator
  Terminator1 : Terminator
  Terminator2 : Terminator
  wires:
  NtcStInfo/1 -> Terminator1/1
  NtcNr/1 -> Terminator/1
  NtcSts/1 -> Data Store Write3/1
  DebStep/1 -> Terminator2/1

== system CF009A_GmOvrlStMgr/GmOvrlStMgr/GmOvrlStMgrInit1/NVM_NOK/CopyRight2 ==

== system CF009A_GmOvrlStMgr/GmOvrlStMgr/GmOvrlStMgrInit1/NVM_Ok/CopyRight2 ==

== system CF009A_GmOvrlStMgr/GmOvrlStMgr/GmOvrlStMgrInit1/Saturate/CopyRight2 ==

== system CF009A_GmOvrlStMgr/GmOvrlStMgr/GmOvrlStMgrInit1/StepDown/CopyRight2 ==

== system CF009A_GmOvrlStMgr/GmOvrlStMgr/GmOvrlStMgrPer1/ApaIntv/CopyRight2 ==

== system CF009A_GmOvrlStMgr/GmOvrlStMgr/GmOvrlStMgrPer1/ApaIntv/If Action Subsystem ==
  In1 : Inport
  Action Port : ActionPort  ActionType=then
  CopyRight2 : Subsystem  Description=|  mask(Copyright Information){none=on}
      | Copyright info block.                                               
      |                                                                     
      | Place copyright information at the top of every subsystem in design.
      mask prompts: none "No parameters"
      mask help: Place copyright information at the top of every subsystem in design.
      mask Display:
      | NxtrConf = 'Nexteer Confidential';
      | 
      | sys = bdroot; %handle for the current model ("system")
      | first = get_param(sys,'Created');
      | first = first(end-3:end);  %year is last four digits
      | 
      | last = get_param(sys,'LastModifiedDate');
      | if isempty(last)
      |     last = datestr(now,'yyyy');
      | else
      |     last = last(end-3:end);
      | end
      | 
      | if strcmp(first,last)
      |     fprintf('%s -- Copyright %s Nexteer',NxtrConf,first)
      | else
      |     fprintf('%s -- %s%s- %s Nexteer',NxtrConf,char(169),first,last)
      | end
  Out1 : Outport
  wires:
  In1/1 -> Out1/1

== system CF009A_GmOvrlStMgr/GmOvrlStMgr/GmOvrlStMgrPer1/ApaIntv/If Action Subsystem1 ==
  In1 : Inport
  Action Port : ActionPort  ActionType=else
  CopyRight2 : Subsystem  Description=|  mask(Copyright Information){none=on}
      | Copyright info block.                                               
      |                                                                     
      | Place copyright information at the top of every subsystem in design.
      mask prompts: none "No parameters"
      mask help: Place copyright information at the top of every subsystem in design.
      mask Display:
      | NxtrConf = 'Nexteer Confidential';
      | 
      | sys = bdroot; %handle for the current model ("system")
      | first = get_param(sys,'Created');
      | first = first(end-3:end);  %year is last four digits
      | 
      | last = get_param(sys,'LastModifiedDate');
      | if isempty(last)
      |     last = datestr(now,'yyyy');
      | else
      |     last = last(end-3:end);
      | end
      | 
      | if strcmp(first,last)
      |     fprintf('%s -- Copyright %s Nexteer',NxtrConf,first)
      | else
      |     fprintf('%s -- %s%s- %s Nexteer',NxtrConf,char(169),first,last)
      | end
  Out1 : Outport
  wires:
  In1/1 -> Out1/1

== system CF009A_GmOvrlStMgr/GmOvrlStMgr/GmOvrlStMgrPer1/ApaIntv/Timer for ApaIntv ==
  Ena : Inport
  TiThd : Inport  Port=2
  Constant : Constant  Value=0  OutDataTypeStr=uint32
  Constant2 : Constant  Value=MILLISECTO100MICROSECCNVN_CNT_U32
  CopyRight2 : Subsystem  Description=|  mask(Copyright Information){none=on}
      | Copyright info block.                                               
      |                                                                     
      | Place copyright information at the top of every subsystem in design.
      mask prompts: none "No parameters"
      mask help: Place copyright information at the top of every subsystem in design.
      mask Display:
      | NxtrConf = 'Nexteer Confidential';
      | 
      | sys = bdroot; %handle for the current model ("system")
      | first = get_param(sys,'Created');
      | first = first(end-3:end);  %year is last four digits
      | 
      | last = get_param(sys,'LastModifiedDate');
      | if isempty(last)
      |     last = datestr(now,'yyyy');
      | else
      |     last = last(end-3:end);
      | end
      | 
      | if strcmp(first,last)
      |     fprintf('%s -- Copyright %s Nexteer',NxtrConf,first)
      | else
      |     fprintf('%s -- %s%s- %s Nexteer',NxtrConf,char(169),first,last)
      | end
  Data Store Read : DataStoreRead  Priority=1  DataStoreName=PrevApaIntvEna
      settings: AttributesFormatString="Priority:  %<Priority>"
  Data Store Write1 : DataStoreWrite  Priority=2  DataStoreName=PrevApaIntvEna
      settings: AttributesFormatString="Priority:  %<Priority>"
  If : If  NumInputs=2  IfExpression=u1&(~u2)  ElseIfExpressions=u1&u2
  If Action Subsystem : Subsystem  TreatAsAtomicUnit=on
  If Action Subsystem1 : Subsystem  TreatAsAtomicUnit=on
  If Action Subsystem2 : Subsystem  TreatAsAtomicUnit=on
  Merge : Merge  Inputs=3
  Product : Product
  Relational Operator3 : RelationalOperator  OutDataTypeStr=boolean
  Out1 : Outport
  wires:
  If Action Subsystem2/1(Out1) -> Merge/2
  If/2 -> If Action Subsystem2/Action
  Data Store Read/1 -> If/2
  Ena/1 -> If/1, Data Store Write1/1
  Relational Operator3/1 -> Out1/1
  Merge/1 -> Relational Operator3/1
  Product/1 -> Relational Operator3/2
  Constant2/1 -> Product/2
  TiThd/1 -> Product/1
  Constant/1 -> If Action Subsystem1/1(In1)
  If Action Subsystem1/1(Out1) -> Merge/3
  If Action Subsystem/1(Out) -> Merge/1
  If/3 -> If Action Subsystem1/Action
  If/1 -> If Action Subsystem/Action

== system CF009A_GmOvrlStMgr/GmOvrlStMgr/GmOvrlStMgrPer1/HaptcStTransActvToWaitFlg/CopyRight2 ==

== system CF009A_GmOvrlStMgr/GmOvrlStMgr/GmOvrlStMgrPer1/HaptcStTransActvToWaitFlg/ElpseTi ==
  Action Port : ActionPort  ActionType=then
  Constant : Constant  RequirementInfo={} %GIDa_fa9c206c_9067_4e60_8894_8d33b601da2a  Value=GmOvrlStMgrHaptcDurn
  Constant1 : Constant  Value=MILLISECTO100MICROSECCNVN_CNT_U32
  CopyRight2 : Subsystem  Description=|  mask(Copyright Information){none=on}
      | Copyright info block.                                               
      |                                                                     
      | Place copyright information at the top of every subsystem in design.
      mask prompts: none "No parameters"
      mask help: Place copyright information at the top of every subsystem in design.
      mask Display:
      | NxtrConf = 'Nexteer Confidential';
      | 
      | sys = bdroot; %handle for the current model ("system")
      | first = get_param(sys,'Created');
      | if(isempty(first))
      |     first = datestr(now,'yyyy');
      | else
      |     first = first(end-3:end);  %year is last four digits
      | end
      | 
      | last = get_param(sys,'LastModifiedDate');
      | if isempty(last)
      |     last = datestr(now,'yyyy');
      | else
      |     last = last(end-3:end);
      | end
      | 
      | if strcmp(first,last)
      |     fprintf('%s -- Copyright %s Nexteer',NxtrConf,first)
      | else
      |     fprintf('%s -- %s%s- %s Nexteer',NxtrConf,char(169),first,last)
      | end
  Data Store Read : DataStoreRead  DataStoreName=HaptcStTranActvToWaitRefTi
  GetTiSpan100MicroSec32bit : Subsystem
  If4 : If  IfExpression=u1
  Merge1 : Merge
  Product1 : Product
  Relational Operator : RelationalOperator  OutDataTypeStr=boolean
  Set False Subsystem : Subsystem  TreatAsAtomicUnit=on
  Set True Subsystem : Subsystem  TreatAsAtomicUnit=on
  Out1 : Outport
  wires:
  Constant/1 -> Product1/1
  Product1/1 -> Relational Operator/2
  Constant1/1 -> Product1/2
  If4/2 -> Set False Subsystem/Action
  Set False Subsystem/1(Out1) -> Merge1/2
  Set True Subsystem/1(Out1) -> Merge1/1
  If4/1 -> Set True Subsystem/Action
  Relational Operator/1 -> If4/1
  GetTiSpan100MicroSec32bit/1(TiSpan) -> Relational Operator/1
  Merge1/1 -> Out1/1
  Data Store Read/1 -> GetTiSpan100MicroSec32bit/1(RefTmr)

== system CF009A_GmOvrlStMgr/GmOvrlStMgr/GmOvrlStMgrPer1/HaptcStTransActvToWaitFlg/RefTi ==
  Action Port : ActionPort  ActionType=else
  Constant13 : Constant  RequirementInfo={} %GIDa_062cf54a_a051_4534_8b9b_47c7f4969e08  Value=false  OutDataTypeStr=boolean
      settings: AttributesFormatString=%<OutDataTypeStr>
  CopyRight2 : Subsystem  Description=|  mask(Copyright Information){none=on}
      | Copyright info block.                                               
      |                                                                     
      | Place copyright information at the top of every subsystem in design.
      mask prompts: none "No parameters"
      mask help: Place copyright information at the top of every subsystem in design.
      mask Display:
      | NxtrConf = 'Nexteer Confidential';
      | 
      | sys = bdroot; %handle for the current model ("system")
      | first = get_param(sys,'Created');
      | if(isempty(first))
      |     first = datestr(now,'yyyy');
      | else
      |     first = first(end-3:end);  %year is last four digits
      | end
      | 
      | last = get_param(sys,'LastModifiedDate');
      | if isempty(last)
      |     last = datestr(now,'yyyy');
      | else
      |     last = last(end-3:end);
      | end
      | 
      | if strcmp(first,last)
      |     fprintf('%s -- Copyright %s Nexteer',NxtrConf,first)
      | else
      |     fprintf('%s -- %s%s- %s Nexteer',NxtrConf,char(169),first,last)
      | end
  Data Store Write9 : DataStoreWrite  DataStoreName=HaptcStTranActvToWaitRefTi
  GetRefTmr100MicroSec32bit : Subsystem
  Out1 : Outport
  wires:
  Constant13/1 -> Out1/1
  GetRefTmr100MicroSec32bit/1(RefTmr) -> Data Store Write9/1

== system CF009A_GmOvrlStMgr/GmOvrlStMgr/GmOvrlStMgrPer1/HwAgServo/CopyRight2 ==

== system CF009A_GmOvrlStMgr/GmOvrlStMgr/GmOvrlStMgrPer1/HwAgServo/If Action Subsystem ==
  ApaSt : Inport
  HwAgTraj : Inport  Port=2
  Action Port : ActionPort  ActionType=then
  ApaStatusActive : Subsystem  TreatAsAtomicUnit=on
  ApaStatusNotActive : Subsystem  TreatAsAtomicUnit=on
  Constant : Constant  Value=APASTACTV_CNT_U08
  CopyRight2 : Subsystem  Description=|  mask(Copyright Information){none=on}
      | Copyright info block.                                               
      |                                                                     
      | Place copyright information at the top of every subsystem in design.
      mask prompts: none "No parameters"
      mask help: Place copyright information at the top of every subsystem in design.
      mask Display:
      | NxtrConf = 'Nexteer Confidential';
      | 
      | sys = bdroot; %handle for the current model ("system")
      | first = get_param(sys,'Created');
      | if(isempty(first))
      |     first = datestr(now,'yyyy');
      | else
      |     first = first(end-3:end);  %year is last four digits
      | end
      | 
      | last = get_param(sys,'LastModifiedDate');
      | if isempty(last)
      |     last = datestr(now,'yyyy');
      | else
      |     last = last(end-3:end);
      | end
      | 
      | if strcmp(first,last)
      |     fprintf('%s -- Copyright %s Nexteer',NxtrConf,first)
      | else
      |     fprintf('%s -- %s%s- %s Nexteer',NxtrConf,char(169),first,last)
      | end
  If : If  NumInputs=2  IfExpression=u1 == u2
  Merge : Merge
  Merge1 : Merge
  HwAgServoEna : Outport
  HwAgServoCmd : Outport  Port=2
  wires:
  ApaSt/1 -> If/1
  Constant/1 -> If/2
  If/1 -> ApaStatusActive/Action
  If/2 -> ApaStatusNotActive/Action
  ApaStatusActive/2(HwAgServoCmd) -> Merge/1
  ApaStatusNotActive/1(HwAgServoCmd) -> Merge/2
  Merge/1 -> HwAgServoCmd/1
  ApaStatusActive/1(HwAgServoEna) -> Merge1/1
  ApaStatusNotActive/2(HwAgServoEna) -> Merge1/2
  Merge1/1 -> HwAgServoEna/1
  HwAgTraj/1 -> ApaStatusNotActive/1(HwAgTraj)

== system CF009A_GmOvrlStMgr/GmOvrlStMgr/GmOvrlStMgrPer1/HwAgServo/If Action Subsystem1 ==
  ApaSt : Inport
  HwAgTarLimd : Inport  Port=2
  Action Port : ActionPort  ActionType=else
  ApaStatusActive : Subsystem  TreatAsAtomicUnit=on
  ApaStatusNotActive : Subsystem  TreatAsAtomicUnit=on
  Constant : Constant  Value=APASTACTV_CNT_U08
  CopyRight2 : Subsystem  Description=|  mask(Copyright Information){none=on}
      | Copyright info block.                                               
      |                                                                     
      | Place copyright information at the top of every subsystem in design.
      mask prompts: none "No parameters"
      mask help: Place copyright information at the top of every subsystem in design.
      mask Display:
      | NxtrConf = 'Nexteer Confidential';
      | 
      | sys = bdroot; %handle for the current model ("system")
      | first = get_param(sys,'Created');
      | if(isempty(first))
      |     first = datestr(now,'yyyy');
      | else
      |     first = first(end-3:end);  %year is last four digits
      | end
      | 
      | last = get_param(sys,'LastModifiedDate');
      | if isempty(last)
      |     last = datestr(now,'yyyy');
      | else
      |     last = last(end-3:end);
      | end
      | 
      | if strcmp(first,last)
      |     fprintf('%s -- Copyright %s Nexteer',NxtrConf,first)
      | else
      |     fprintf('%s -- %s%s- %s Nexteer',NxtrConf,char(169),first,last)
      | end
  If : If  NumInputs=2  IfExpression=u1 == u2
  Merge : Merge
  Merge1 : Merge
  HwAgServoCmd : Outport
  HwAgServoEna : Outport  Port=2
  wires:
  ApaSt/1 -> If/1
  Constant/1 -> If/2
  If/1 -> ApaStatusActive/Action
  If/2 -> ApaStatusNotActive/Action
  Merge/1 -> HwAgServoCmd/1
  Merge1/1 -> HwAgServoEna/1
  HwAgTarLimd/1 -> ApaStatusActive/1(HwAgTarLimd)
  ApaStatusActive/1(HwAgServoCmd) -> Merge/1
  ApaStatusNotActive/2(HwAgServoCmd) -> Merge/2
  ApaStatusNotActive/1(HwAgServoEna) -> Merge1/2
  ApaStatusActive/2(HwAgServoEna) -> Merge1/1

== system CF009A_GmOvrlStMgr/GmOvrlStMgr/GmOvrlStMgrPer1/HwAgTarLimiter/CopyRight2 ==

== system CF009A_GmOvrlStMgr/GmOvrlStMgr/GmOvrlStMgrPer1/HwTqFildIntlChk/CopyRight2 ==

== system CF009A_GmOvrlStMgr/GmOvrlStMgr/GmOvrlStMgrPer1/Inct_IgnCntr_Once/CopyRight2 ==
